simulink model "Global_MPC"  (R2023b)
settings: Solver=FixedStepAuto  StartTime=0.0  StopTime=3600  FixedStep=3600  RelTol=1e-3
values from neighbouring files (symbols this model uses):
  c = standardConstants    [Run_simulation.m]
settings Model: Creator=is123  LastModifiedBy=is123

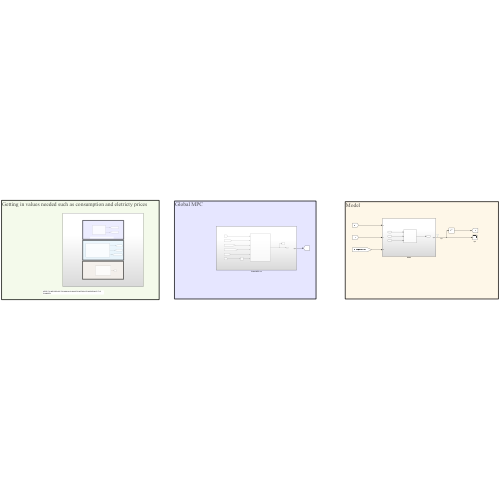
[thumbnail: Simulink's stored preview of the top-level diagram]
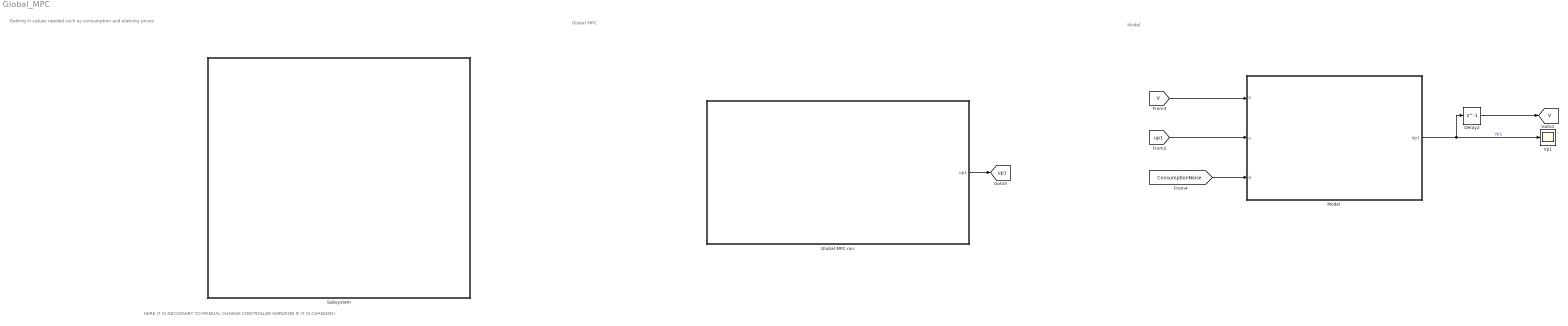
== system Global_MPC ==
  note: Getting in values needed such as consumption and eletricty prices
  note: Global MPC
  note: Model
  note: HERE IT IS NECCESARY TO MANUAL CHANGE CONTROLLER HORIZION IF IT IS CHANGED!
  Delay2 : Delay  DelayLength=1  InitialCondition=c.V
  Global MPC run : Subsystem
  Model : Subsystem
  Subsystem : Subsystem
  Vp1 : Scope
  tag scope: V=global, up1=global
  wires:
  Model/1(Vp1) -> Delay2/1, Vp1/1  "Vp1"
  [V] -> Model/1(V)
  Delay2/1 -> [V]
  [up1] -> Model/2(u)
  [ConsumptionNoise] -> Model/3(d)
  Global MPC run/1(up1) -> [up1]

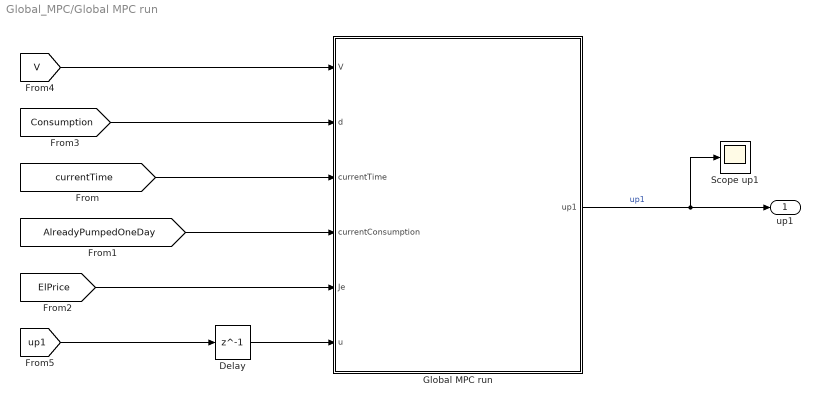
== system Global_MPC/Global MPC run ==
  Delay : Delay  DelayLength=1  InitialCondition=[0;0;0]
  Global MPC run : MATLAB Function  TreatAsAtomicUnit=on
  Scope up1 : Scope
  up1 : Outport
  wires:
  [currentTime] -> Global MPC run/3(currentTime)
  [AlreadyPumpedOneDay] -> Global MPC run/4(currentConsumption)
  [ElPrice] -> Global MPC run/5(Je)
  Global MPC run/1(up1) -> up1/1, Scope up1/1  "up1"
  Delay/1 -> Global MPC run/6(u)
  [Consumption] -> Global MPC run/2(d)
  [V] -> Global MPC run/1(V)
  [up1] -> Delay/1

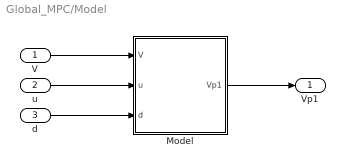
== system Global_MPC/Model ==
  V : Inport
  u : Inport  Port=2
  d : Inport  Port=3
  Model : MATLAB Function  TreatAsAtomicUnit=on
  Vp1 : Outport
  wires:
  Model/1(Vp1) -> Vp1/1
  V/1 -> Model/1(V)
  u/1 -> Model/2(u)
  d/1 -> Model/3(d)

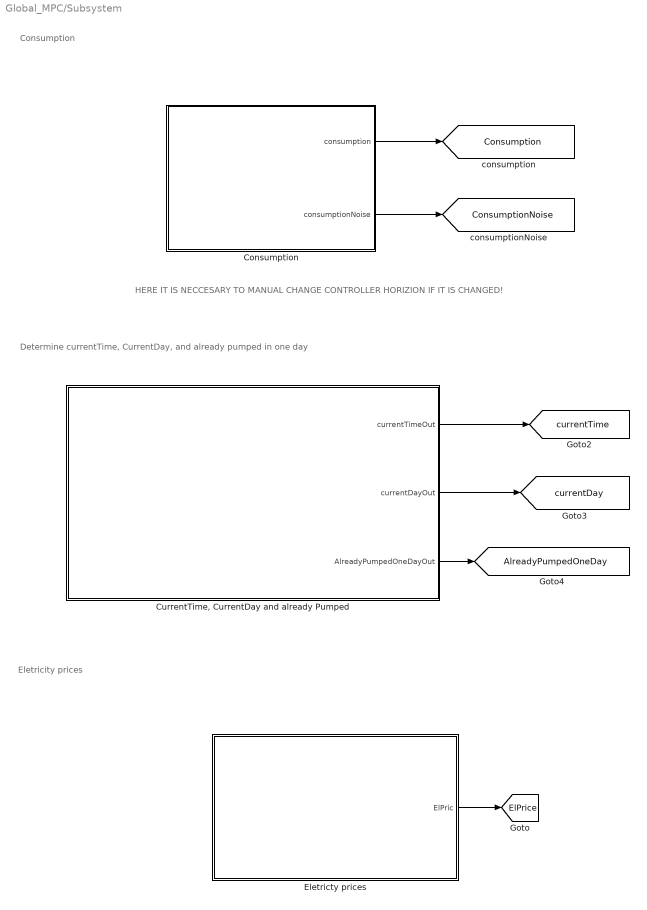
== system Global_MPC/Subsystem ==
  note: HERE IT IS NECCESARY TO MANUAL CHANGE CONTROLLER HORIZION IF IT IS CHANGED!
  note: Determine currentTime, CurrentDay, and already pumped in one day
  note: Consumption
  note: Eletricity prices
  Consumption : Subsystem
  "CurrentTime, CurrentDay and already Pumped" : Subsystem
  Eletricty prices : Subsystem
  tag scope: AlreadyPumpedOneDay=global, Consumption=global, ConsumptionNoise=global, ElPrice=global, currentDay=global, currentTime=global
  wires:
  Eletricty prices/1(ElPric) -> [ElPrice]
  "CurrentTime, CurrentDay and already Pumped"/3(AlreadyPumpedOneDayOut) -> [AlreadyPumpedOneDay]
  "CurrentTime, CurrentDay and already Pumped"/1(currentTimeOut) -> [currentTime]
  Consumption/1(consumption) -> [Consumption]
  Consumption/2(consumptionNoise) -> [ConsumptionNoise]
  "CurrentTime, CurrentDay and already Pumped"/2(currentDayOut) -> [currentDay]

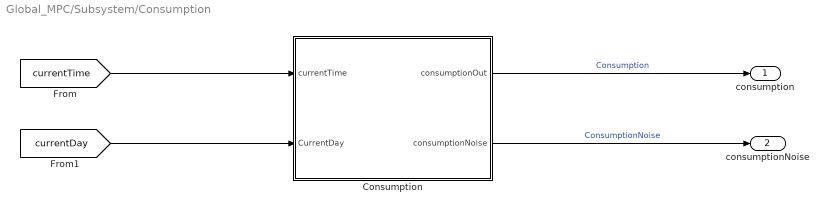
== system Global_MPC/Subsystem/Consumption ==
  Consumption : MATLAB Function  TreatAsAtomicUnit=on
  consumption : Outport
  consumptionNoise : Outport  Port=2
  wires:
  Consumption/1(consumptionOut) -> consumption/1  "Consumption"
  [currentTime] -> Consumption/1(currentTime)
  [currentDay] -> Consumption/2(CurrentDay)
  Consumption/2(consumptionNoise) -> consumptionNoise/1  "ConsumptionNoise"

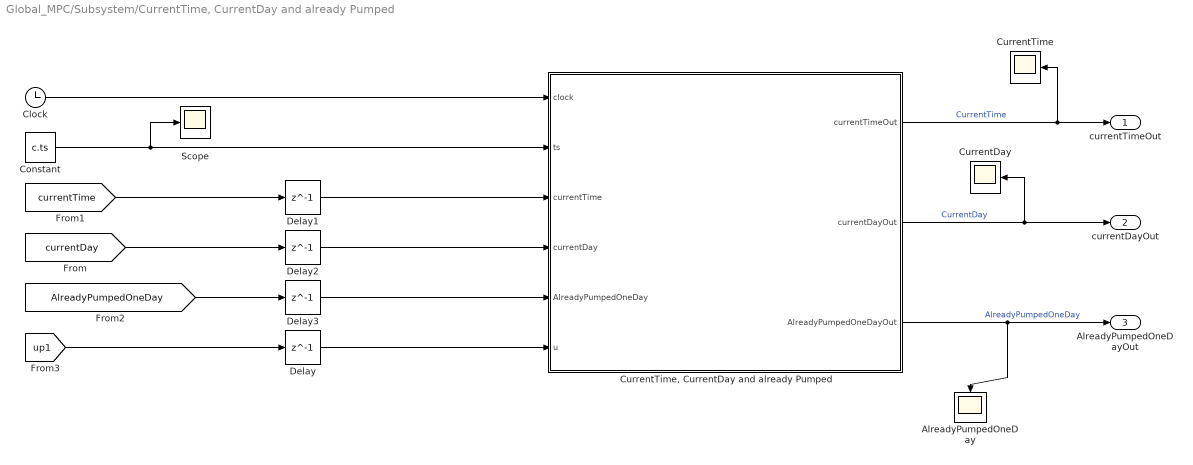
== system Global_MPC/Subsystem/CurrentTime, CurrentDay and already Pumped ==
  AlreadyPumpedOneDay : Scope
  Clock : Clock
  Constant : Constant  Value=c.ts
  CurrentDay : Scope
  CurrentTime : Scope
  "CurrentTime, CurrentDay and already Pumped" : MATLAB Function  TreatAsAtomicUnit=on
  Delay : Delay  DelayLength=1  InitialCondition=[0;0;0]
  Delay1 : Delay  DelayLength=1  InitialCondition=0
  Delay2 : Delay  DelayLength=1  InitialCondition=0
  Delay3 : Delay  DelayLength=1  InitialCondition=[0;0;0]
  Scope : Scope
  currentTimeOut : Outport
  currentDayOut : Outport  Port=2
  AlreadyPumpedOneDayOut : Outport  Port=3
  wires:
  "CurrentTime, CurrentDay and already Pumped"/2(currentDayOut) -> currentDayOut/1, CurrentDay/1  "CurrentDay"
  [currentDay] -> Delay2/1
  "CurrentTime, CurrentDay and already Pumped"/1(currentTimeOut) -> currentTimeOut/1, CurrentTime/1  "CurrentTime"
  Delay3/1 -> "CurrentTime, CurrentDay and already Pumped"/5(AlreadyPumpedOneDay)
  Delay2/1 -> "CurrentTime, CurrentDay and already Pumped"/4(currentDay)
  "CurrentTime, CurrentDay and already Pumped"/3(AlreadyPumpedOneDayOut) -> AlreadyPumpedOneDayOut/1, AlreadyPumpedOneDay/1  "AlreadyPumpedOneDay"
  Delay1/1 -> "CurrentTime, CurrentDay and already Pumped"/3(currentTime)
  [currentTime] -> Delay1/1
  [AlreadyPumpedOneDay] -> Delay3/1
  [up1] -> Delay/1
  Clock/1 -> "CurrentTime, CurrentDay and already Pumped"/1(clock)
  Delay/1 -> "CurrentTime, CurrentDay and already Pumped"/6(u)
  Constant/1 -> Scope/1, "CurrentTime, CurrentDay and already Pumped"/2(ts)

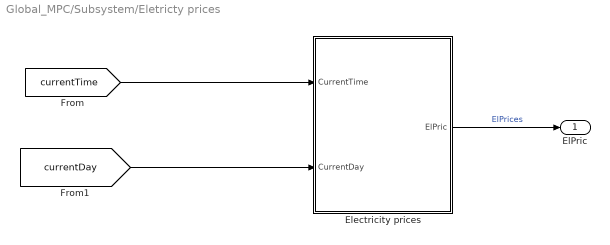
== system Global_MPC/Subsystem/Eletricty prices ==
  Electricity prices : MATLAB Function  TreatAsAtomicUnit=on
  ElPric : Outport
  wires:
  [currentTime] -> Electricity prices/1(CurrentTime)
  [currentDay] -> Electricity prices/2(CurrentDay)
  Electricity prices/1(ElPric) -> ElPric/1  "ElPrices"

== matlab function Global_MPC/Subsystem/Consumption/Consumption ==
  data: currentTime input; consumptionOut output; consumptionNoise output; CurrentDay input
function [consumptionOut,consumptionNoise]  = consumption(currentTime,CurrentDay)
%Getting the consumption for MPC and model 
coder.extrinsic('consumption')

%Setting zeros because simulink needs it
consumptionNoise=zeros(1,1); 
%zeros(Nc,1) Nc needed to be updated if changes 
consumptionOut=zeros(24,1); 

%Calling the consumption to get the consumptions needed 
[consumptionOut,consumptionNoiseTemp]=consumption(currentTime,CurrentDay); 
%For the model only the first consumption is neccesary! 
consumptionNoise=consumptionNoiseTemp(1,1); 
end

== matlab function Global_MPC/Model/Model ==
  data: V input; u input; Vp1 output; d input
function Vp1 = model(V,u,d)
%Caling the model function


%coder.extrinsic('Model')
%Setting the output to zero becuase it is needed
Vp1=zeros(1,1); 
%calling the model function to get the next volumen
Vp1=Model(V,u,d);

== matlab function Global_MPC/Subsystem/CurrentTime, CurrentDay and already Pumped/CurrentTime, CurrentDay and already Pumped ==
  data: clock input; ts input; currentTimeOut output; currentTime input; currentDay input; AlreadyPumpedOneDay input; currentDayOut output; AlreadyPumpedOneDayOut output; u input
% Small function used to determine the time of day and what day it is
% furthermore it keeps track of how much have pump in a day 
function [currentTimeOut, currentDayOut,AlreadyPumpedOneDayOut] = currentTime(clock,ts, currentTime,currentDay,AlreadyPumpedOneDay,u)
%Defining amount of seconds per day
SecondsPerDay=24*3600;

if clock==0 % Making sure that the simulation starts from 0 
    currentTimeOut=0; 
else %Add the sample time to the last currentTime to update the time
    currentTimeOut=currentTime+3600*ts; 
end 
%If more than a day haves gone by add one to current day, set AlreadyPump
%to zero and current to zero, otherwise same current day and update the
%amount pump in one day! 
 if currentTimeOut>=SecondsPerDay
     currentDayOut=currentDay+1;
     AlreadyPumpedOneDayOut=zeros(3,1); 
     currentTimeOut=0; 
 else 
     currentDayOut=currentDay; 
     AlreadyPumpedOneDayOut=AlreadyPumpedOneDay+ts*u; 
 end 

end

== matlab function Global_MPC/Subsystem/Eletricty prices/Electricity prices ==
  data: CurrentTime input; ElPric output; CurrentDay input
function ElPric = ElPrices(CurrentTime,CurrentDay)
%Setting up out because I thin Simulink needs it 
ElPric=zeros(24,1); 
%Calling matlab function to get the electricty price
ElPric=ElectrictyPrices(CurrentTime,CurrentDay);
end

== matlab function Global_MPC/Global MPC run/Global MPC run ==
  data: V input; d input; currentTime input; currentConsumption input; Je input; u input; up1 output
function up1 = RunMPC(V,d,currentTime,currentConsumption, Je,u)
%needed to make the function run 
coder.extrinsic('mpcRun')

%Need to setup the output of the function 
up1=zeros(3,1);

%solving the global model control problem 
[up1,uAll]=mpcRun(V,d,currentTime,currentConsumption, Je,u); 

%Showning time becuase I can! 
disp(currentTime)
end
